simulink library "SimCoreLib"  (R2016b)
settings: Solver=VariableStepAuto  StartTime=0.0  StopTime=10.0  RelTol=1e-3
values from neighbouring files (symbols this model uses):
  Env =     [UAV_modelconfig.mat]
undefined symbols (not defined in the file or in its folder): HDBK, Light, MIL, Sim
undefined symbols (not defined in the file): AC, TrimCondition
libraries: OpenFlightUtilLib x18, SimCoreLib x7, aerolibwind2 x2, aerolib6dofsys x2, aerolibatmos2 x1, aerolibutil x1, aerolib6dof2 x1, aerolibgravity2 x1, aerolibobsolete x1, simulink x1
settings Model: Creator=UAVLAB  LastModifiedBy=rega0051

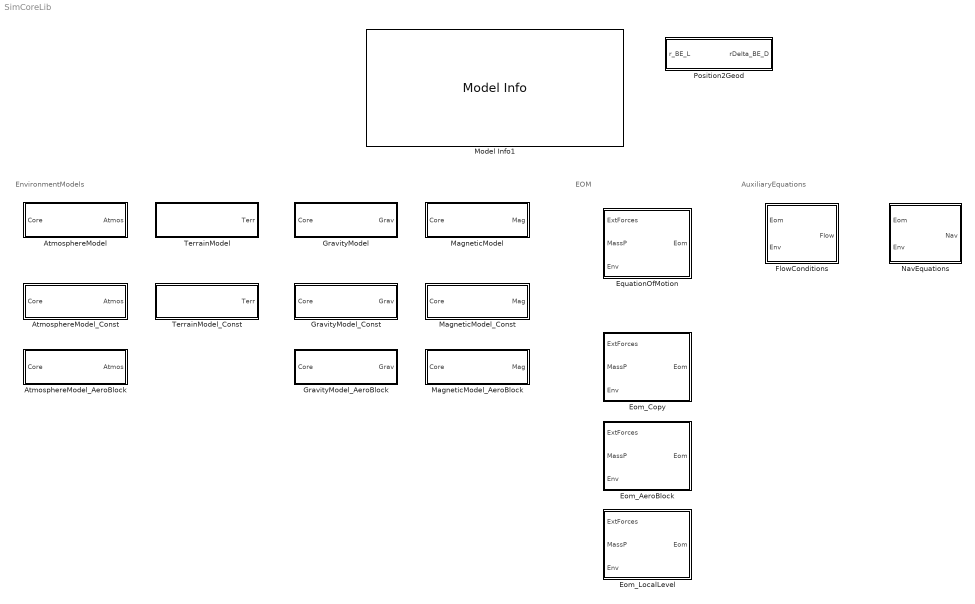
== system SimCoreLib ==
  note: EnvironmentModels
  note: EOM
  note: AuxiliaryEquations
  AtmosphereModel : Subsystem  BlockChoice=AtmosphereModel_AeroBlock
      settings: AttributesFormatString=%<BlockChoice>  TemplateBlock=self  MemberBlocks=AtmosphereModel_AeroBlock,AtmosphereModel_Const
  AtmosphereModel_AeroBlock : Subsystem
  AtmosphereModel_Const : Subsystem
  Eom_AeroBlock : Subsystem  mask(6DoF EoM (Body Axis)){units=Metric (MKS), mtype=Fixed, rep=Euler Angles, xme_0=TrimCondition.InertialIni, Vm_0=TrimCondition.VelocitiesIni, eul_0=TrimCondition.AttitudeIni, pm_0=TrimCondition.RatesIni, mass_0=AC.MassP.mass_kg, mass_e=0.5, mass_f=2.0, inertia=AC.MassP.I_B_kgm2, inertia_e=eye(3), inertia_f=2*eye(3), k_quat=1.0}
      mask prompts: mtype "Mass type:"; rep "Representation:"; xme_0 "Initial position in inertial axes [Xe,Ye,Ze]:"; Vm_0 "Initial velocity in body axes [U,v,w]:"; eul_0 "Initial Euler orientation [roll, pitch, yaw]:"; pm_0 "Initial body rotation rates [p,q,r]:"; mass_0 "Initial mass:"; mass_e "Empty mass:"; mass_f "Full mass:"; inertia_e "Empty inertia matrix:"; inertia_f "Full inertia matrix:"; k_quat "Gain for quaternion normalization:"
      mask help:
      | Integrate the six-degrees-of-freedom equations of motion in body axis.
      |
      | This block has been modified from the original Aerospace Blockset
      | implementation. The inertial position vector (Xe) is no longer computed.
      | The original block did not have a way to add steady state winds to the
      | inertial velocities (Ve) prior to integrating to get Xe. Therefore, this
      | step is performed in the Auxiliary Equations block.
      mask Help: eval('asbhelp(''sixdof_euler_angles'')');
      mask TypeOptions units: Metric (MKS) | English (Velocity in ft/s) | English (Velocity in kts)
      mask TypeOptions mtype: Fixed | Simple Variable | Custom Variable
      mask Callback mtype: aeroicon('aeroblk6dofbody');
      mask TypeOptions rep: Euler Angles | Quaternion
      mask Callback rep: aeroicon('aeroblk6dofbody');
  Eom_Copy : Subsystem
  Eom_LocalLevel : Subsystem
      settings: MinAlgLoopOccurrences=on
  EquationOfMotion : Subsystem  BlockChoice=Eom_AeroBlock
      settings: AttributesFormatString=%<BlockChoice>  TemplateBlock=self  MemberBlocks=Eom_AeroBlock,Eom_Copy,Eom_LocalLevel
  FlowConditions : Subsystem
  GravityModel : Subsystem  BlockChoice=GravityModel_AeroBlock
      settings: AttributesFormatString=%<BlockChoice>  TemplateBlock=self  MemberBlocks=GravityModel_AeroBlock,GravityModel_Const
  GravityModel_AeroBlock : Subsystem
  GravityModel_Const : Subsystem
  MagneticModel : Subsystem  BlockChoice=MagneticModel_AeroBlock
      settings: AttributesFormatString=%<BlockChoice>  TemplateBlock=self  MemberBlocks=MagneticModel_AeroBlock,MagneticModel_Const
  MagneticModel_AeroBlock : Subsystem
  MagneticModel_Const : Subsystem
  Model Info1 : simulink/Model-Wide Utilities/Model Info  Frame=on  DisplayStringWithTags=|  HorizontalTextAlignment=Left  LeftAlignmentValue=0.02  SourceBlockDiagram=SimCoreLib  TagMaxNumber=20
      | MODEL INFORMATION
      | Simulation Core Library (%<ModelName>)
      | 
      | University of Minnesota
      | Aerospace Engineering and Mechanics
      | Copyright 2017 Regents of the University of Minnesota. All rights reserved.
      | 
      | == Update Info ==
      | Last modified by %<LastModifiedBy> on %<LastModificationDate>
  NavEquations : Subsystem
  Position2Geod : Subsystem
  TerrainModel : Subsystem  BlockChoice=TerrainModel_Const
      settings: AttributesFormatString=%<BlockChoice>  TemplateBlock=self  MemberBlocks=TerrainModel_Const
  TerrainModel_Const : Subsystem

== system SimCoreLib/AtmosphereModel ==
  Core : Inport
  AtmosphereModel_AeroBlock : SimCoreLib/AtmosphereModel_AeroBlock
  Atmos : Outport
  wires:
  Core/1 -> AtmosphereModel_AeroBlock/1
  AtmosphereModel_AeroBlock/1 -> Atmos/1

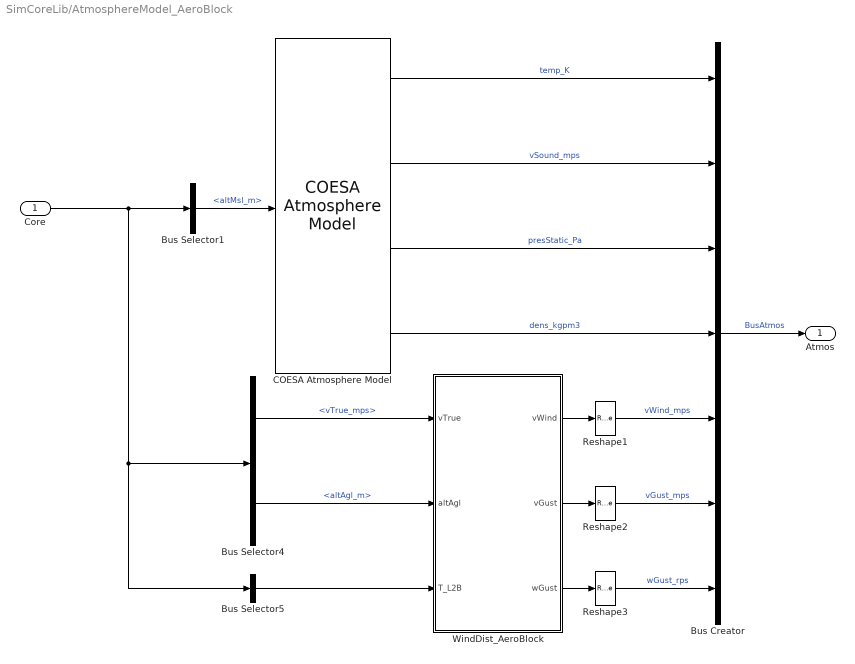
== system SimCoreLib/AtmosphereModel_AeroBlock ==
  Core : Inport
  Bus Creator : BusCreator  Inputs=7  OutDataTypeStr=Bus: BusAtmos
      settings: AttributesFormatString=%<OutDataTypeStr>
  Bus Selector1 : BusSelector  OutputSignals=BusAux.BusNav.altMsl_m
  Bus Selector4 : BusSelector  OutputSignals=BusAux.BusFlow.vTrue_mps,BusAux.BusNav.altAgl_m
  Bus Selector5 : BusSelector  OutputSignals=BusEom.T_L2B  OutputAsBus=on
  COESA Atmosphere Model : aerolibatmos2/COESA Atmosphere Model  units=Metric (MKS)  spec=1976 COESA-extended U.S. Standard Atmosphere  model=Profile  profile_var=High temperature  profile_percent=1%  profile_alt=5 km (16404 ft)  envelope_var=High temperature  envelope_percent=1%  action=Warning
  Reshape1 : Reshape  OutputDimensionality=Column vector (2-D)  OutputDimensions=[3,1]
  Reshape2 : Reshape  OutputDimensionality=Column vector (2-D)  OutputDimensions=[3,1]
  Reshape3 : Reshape  OutputDimensionality=Column vector (2-D)  OutputDimensions=[3,1]
  WindDist_AeroBlock : Subsystem
  Atmos : Outport
  wires:
  Reshape3/1 -> Bus Creator/7  "wGust_rps"
  Reshape2/1 -> Bus Creator/6  "vGust_mps"
  Reshape1/1 -> Bus Creator/5  "vWind_mps"
  WindDist_AeroBlock/1(vWind) -> Reshape1/1
  WindDist_AeroBlock/3(wGust) -> Reshape3/1
  WindDist_AeroBlock/2(vGust) -> Reshape2/1
  Bus Selector1/1 -> COESA Atmosphere Model/1  "<altMsl_m>"
  Bus Selector5/1 -> WindDist_AeroBlock/3(T_L2B)
  Bus Selector4/1 -> WindDist_AeroBlock/1(vTrue)  "<vTrue_mps>"
  COESA Atmosphere Model/4 -> Bus Creator/4  "dens_kgpm3"
  COESA Atmosphere Model/3 -> Bus Creator/3  "presStatic_Pa"
  COESA Atmosphere Model/2 -> Bus Creator/2  "vSound_mps"
  COESA Atmosphere Model/1 -> Bus Creator/1  "temp_K"
  Core/1 -> Bus Selector1/1, Bus Selector4/1, Bus Selector5/1
  Bus Creator/1 -> Atmos/1  "BusAtmos"
  Bus Selector4/2 -> WindDist_AeroBlock/2(altAgl)  "<altAgl_m>"

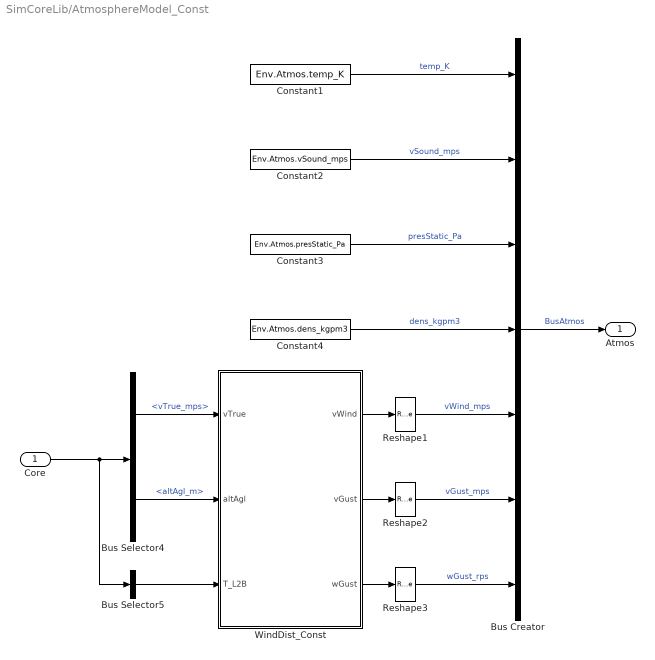
== system SimCoreLib/AtmosphereModel_Const ==
  Core : Inport
  Bus Creator : BusCreator  Inputs=7  OutDataTypeStr=Bus: BusAtmos
      settings: AttributesFormatString=%<OutDataTypeStr>
  Bus Selector4 : BusSelector  OutputSignals=BusAux.BusFlow.vTrue_mps,BusAux.BusNav.altAgl_m
  Bus Selector5 : BusSelector  OutputSignals=BusEom.T_L2B  OutputAsBus=on
  Constant1 : Constant  Value=Env.Atmos.temp_K
      settings: AttributesFormatString=%<Value>
  Constant2 : Constant  Value=Env.Atmos.vSound_mps
      settings: AttributesFormatString=%<Value>
  Constant3 : Constant  Value=Env.Atmos.presStatic_Pa
      settings: AttributesFormatString=%<Value>
  Constant4 : Constant  Value=Env.Atmos.dens_kgpm3
      settings: AttributesFormatString=%<Value>
  Reshape1 : Reshape  OutputDimensionality=Column vector (2-D)  OutputDimensions=[3,1]
  Reshape2 : Reshape  OutputDimensionality=Column vector (2-D)  OutputDimensions=[3,1]
  Reshape3 : Reshape  OutputDimensionality=Column vector (2-D)  OutputDimensions=[3,1]
  WindDist_Const : Subsystem
      settings: MinAlgLoopOccurrences=on
  Atmos : Outport
  wires:
  Reshape3/1 -> Bus Creator/7  "wGust_rps"
  Reshape2/1 -> Bus Creator/6  "vGust_mps"
  Reshape1/1 -> Bus Creator/5  "vWind_mps"
  Bus Creator/1 -> Atmos/1  "BusAtmos"
  Core/1 -> Bus Selector5/1, Bus Selector4/1
  Constant1/1 -> Bus Creator/1  "temp_K"
  WindDist_Const/1(vWind) -> Reshape1/1
  WindDist_Const/3(wGust) -> Reshape3/1
  Constant2/1 -> Bus Creator/2  "vSound_mps"
  Constant3/1 -> Bus Creator/3  "presStatic_Pa"
  WindDist_Const/2(vGust) -> Reshape2/1
  Constant4/1 -> Bus Creator/4  "dens_kgpm3"
  Bus Selector4/1 -> WindDist_Const/1(vTrue)  "<vTrue_mps>"
  Bus Selector4/2 -> WindDist_Const/2(altAgl)  "<altAgl_m>"
  Bus Selector5/1 -> WindDist_Const/3(T_L2B)

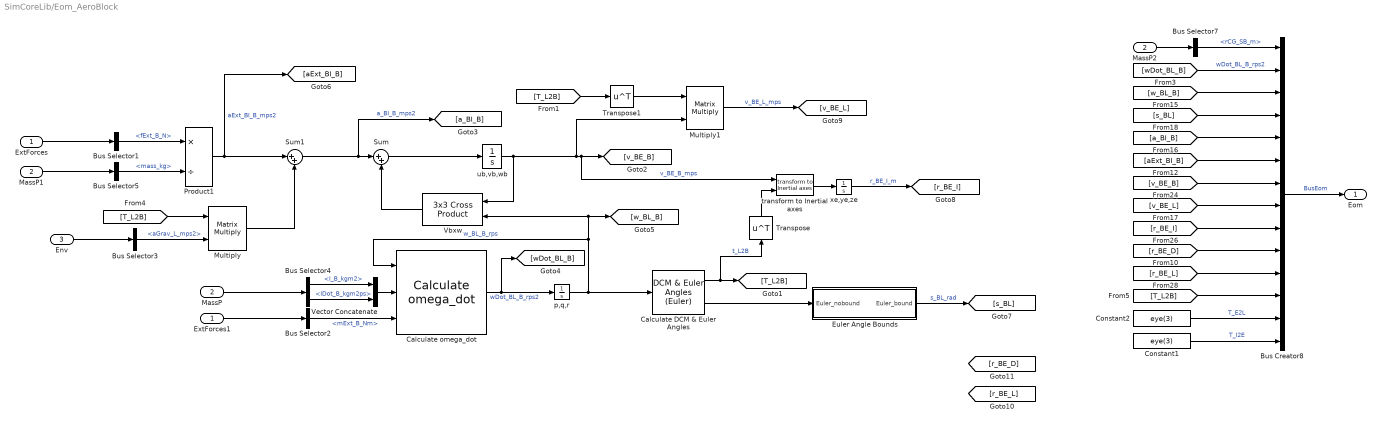
== system SimCoreLib/Eom_AeroBlock ==
  ExtForces : Inport
  MassP : Inport  Port=2
  Env : Inport  Port=3
  Bus Selector1 : BusSelector  OutputSignals=fExt_B_N
  Bus Selector2 : BusSelector  OutputSignals=mExt_B_Nm
  Bus Selector3 : BusSelector  OutputSignals=BusGrav.aGrav_L_mps2
  Bus Selector4 : BusSelector  OutputSignals=I_B_kgm2,IDot_B_kgm2ps
  Bus Selector5 : BusSelector  OutputSignals=mass_kg
  Bus Selector7 : BusSelector  OutputSignals=rCG_SB_m
  Bus Creator8 : BusCreator  Inputs=14  OutDataTypeStr=Bus: BusEom
      settings: AttributesFormatString=%<OutDataTypeStr>
  Calculate DCM & Euler Angles : aerolib6dofsys/DCM & Euler Angles (Euler)  SystemSampleTime=-1
  Calculate omega_dot : aerolib6dofsys/Calculate omega_dot  SystemSampleTime=-1
  Constant1 : Constant  Value=eye(3)
      settings: AttributesFormatString=%<Value>
  Constant2 : Constant  Value=eye(3)
      settings: AttributesFormatString=%<Value>
  Euler Angle Bounds : Subsystem
  ExtForces1 : InportShadow
  MassP1 : InportShadow  Port=2
  MassP2 : InportShadow  Port=2
  Multiply : Product  Multiplication=Matrix(*)  SaturateOnIntegerOverflow=on  InputSameDT=on  OutDataTypeStr=Inherit: Same as first input
  Multiply1 : Product  Multiplication=Matrix(*)  SaturateOnIntegerOverflow=on  InputSameDT=on  OutDataTypeStr=Inherit: Same as first input
  Product1 : Product  Inputs=*/  SaturateOnIntegerOverflow=on  OutDataTypeStr=Inherit: Same as first input
  Sum : Sum  Inputs=|++  SaturateOnIntegerOverflow=on
  Sum1 : Sum  Inputs=|++  SaturateOnIntegerOverflow=on
  Transpose : Math  Operator=transpose  SaturateOnIntegerOverflow=on
  Transpose1 : Math  Operator=transpose  SaturateOnIntegerOverflow=on
  Vbxw : aerolibutil/3x3 Cross Product
  Vector Concatenate : Concatenate  Mode=Multidimensional array
  "p,q,r " : Integrator  InitialCondition=pm_0
  "transform to Inertial axes " : aerolib6dof2/6DOF (Euler Angles)/transform to Inertial axes   SystemSampleTime=-1
  ub,vb,wb : Integrator  InitialCondition=convvel(Vm_0,'m/s','m/s')
  xe,ye,ze : Integrator  InitialCondition=xme_0
  Eom : Outport  OutDataTypeStr=Bus: BusEom
  wires:
  Multiply1/1 -> [v_BE_L]  "v_BE_L_mps"
  [T_L2B] -> Transpose1/1
  Transpose1/1 -> Multiply1/1
  xe,ye,ze/1 -> [r_BE_I]  "r_BE_I_m"
  "transform to Inertial axes "/1 -> xe,ye,ze/1
  Transpose/1 -> "transform to Inertial axes "/2
  Bus Creator8/1 -> Eom/1  "BusEom"
  [T_L2B] -> Bus Creator8/12
  [s_BL] -> Bus Creator8/4
  [a_BI_B] -> Bus Creator8/5
  [r_BE_D] -> Bus Creator8/10
  [w_BL_B] -> Bus Creator8/3
  [aExt_BI_B] -> Bus Creator8/6
  [v_BE_L] -> Bus Creator8/8
  [r_BE_L] -> Bus Creator8/11
  MassP2/1 -> Bus Selector7/1
  Bus Selector7/1 -> Bus Creator8/1  "<rCG_SB_m>"
  [v_BE_B] -> Bus Creator8/7
  [r_BE_I] -> Bus Creator8/9
  Constant1/1 -> Bus Creator8/14  "T_I2E"
  Constant2/1 -> Bus Creator8/13  "T_E2L"
  [wDot_BL_B] -> Bus Creator8/2  "wDot_BL_B_rps2"
  Product1/1 -> Sum1/1, [aExt_BI_B]  "aExt_BI_B_mps2"
  Bus Selector5/1 -> Product1/2  "<mass_kg>"
  MassP1/1 -> Bus Selector5/1
  Vector Concatenate/1 -> Calculate omega_dot/2
  Bus Selector4/1 -> Vector Concatenate/1  "<I_B_kgm2>"
  Bus Selector4/2 -> Vector Concatenate/2  "<IDot_B_kgm2ps>"
  MassP/1 -> Bus Selector4/1
  Bus Selector2/1 -> Calculate omega_dot/3  "<mExt_B_Nm>"
  ExtForces1/1 -> Bus Selector2/1
  Env/1 -> Bus Selector3/1
  Bus Selector3/1 -> Multiply/2  "<aGrav_L_mps2>"
  [T_L2B] -> Multiply/1
  Multiply/1 -> Sum1/2
  Bus Selector1/1 -> Product1/1  "<fExt_B_N>"
  ExtForces/1 -> Bus Selector1/1
  Euler Angle Bounds/1(Euler_bound) -> [s_BL]  "s_BL_rad"
  Calculate DCM & Euler Angles/2 -> Euler Angle Bounds/1(Euler_nobound)
  ub,vb,wb/1 -> Vbxw/1, [v_BE_B], "transform to Inertial axes "/1, Multiply1/2  "v_BE_B_mps"
  Vbxw/1 -> Sum/2
  Sum/1 -> ub,vb,wb/1
  "p,q,r "/1 -> Calculate DCM & Euler Angles/1, Vbxw/2, [w_BL_B], Calculate omega_dot/1  "w_BL_B_rps"
  Sum1/1 -> Sum/1, [a_BI_B]  "a_BI_B_mps2"
  Calculate DCM & Euler Angles/1 -> [T_L2B], Transpose/1  "t_L2B"
  Calculate omega_dot/1 -> "p,q,r "/1, [wDot_BL_B]  "wDot_BL_B_rps2"

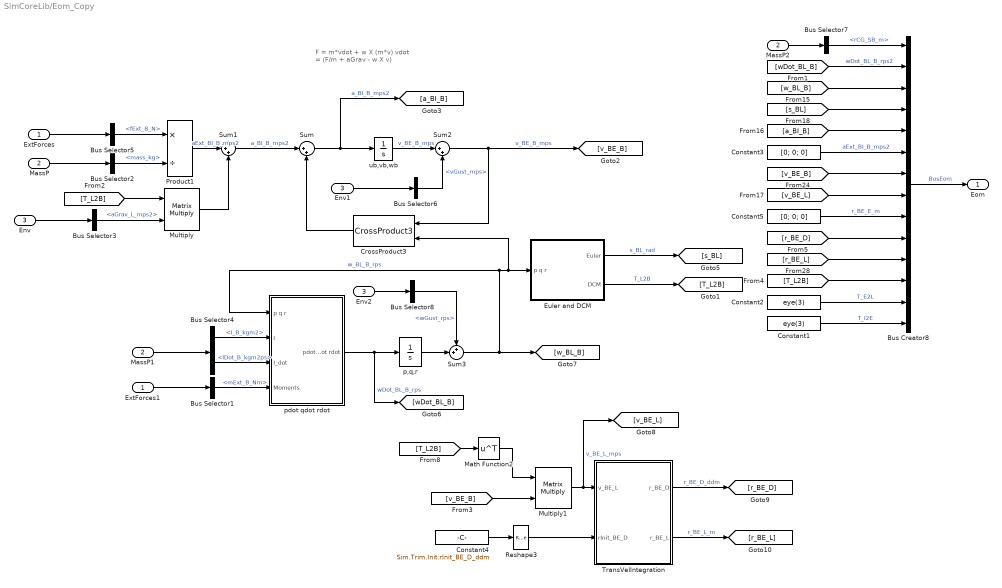
== system SimCoreLib/Eom_Copy ==
  note: F = m*vdot + w X (m*v)
      | vdot = (F/m + aGrav - w X v)
  ExtForces : Inport
  MassP : Inport  Port=2
  Env : Inport  Port=3
  Bus Selector1 : BusSelector  OutputSignals=mExt_B_Nm
  Bus Selector2 : BusSelector  OutputSignals=mass_kg
  Bus Selector3 : BusSelector  OutputSignals=BusGrav.aGrav_L_mps2
  Bus Selector4 : BusSelector  OutputSignals=I_B_kgm2,IDot_B_kgm2ps
  Bus Selector5 : BusSelector  OutputSignals=fExt_B_N
  Bus Selector6 : BusSelector  OutputSignals=BusAtmos.vGust_mps
  Bus Selector7 : BusSelector  OutputSignals=rCG_SB_m
  Bus Selector8 : BusSelector  OutputSignals=BusAtmos.wGust_rps
  Bus Creator8 : BusCreator  Inputs=14  OutDataTypeStr=Bus: BusEom
      settings: AttributesFormatString=%<OutDataTypeStr>
  Constant1 : Constant  Value=eye(3)
      settings: AttributesFormatString=%<Value>
  Constant2 : Constant  Value=eye(3)
      settings: AttributesFormatString=%<Value>
  Constant3 : Constant  Value=[0; 0; 0]
      settings: AttributesFormatString=%<Value>
  Constant4 : Constant  Value=Sim.Trim.Init.rInit_BE_D_ddm
      settings: AttributesFormatString=%<Value>
  Constant5 : Constant  Value=[0; 0; 0]
      settings: AttributesFormatString=%<Value>
  CrossProduct3 : OpenFlightUtilLib/Math/CrossProduct3
  Env1 : InportShadow  Port=3
  Env2 : InportShadow  Port=3
  Euler and DCM : Subsystem
  ExtForces1 : InportShadow
  MassP1 : InportShadow  Port=2
  MassP2 : InportShadow  Port=2
  Math Function2 : Math  Operator=transpose  SaturateOnIntegerOverflow=on
  Multiply : Product  Multiplication=Matrix(*)  SaturateOnIntegerOverflow=on  InputSameDT=on  OutDataTypeStr=Inherit: Same as first input
  Multiply1 : Product  Multiplication=Matrix(*)  SaturateOnIntegerOverflow=on  InputSameDT=on  OutDataTypeStr=Inherit: Same as first input
  Product1 : Product  Inputs=*/  SaturateOnIntegerOverflow=on  OutDataTypeStr=Inherit: Same as first input
  Reshape3 : Reshape  OutputDimensionality=Column vector (2-D)  OutputDimensions=[3,1]
  Sum : Sum  Inputs=|++  SaturateOnIntegerOverflow=on
  Sum1 : Sum  Inputs=|++  SaturateOnIntegerOverflow=on
  Sum2 : Sum  Inputs=|++
  Sum3 : Sum  Inputs=++|
  TransVelIntegration : Subsystem
  "p,q,r " : Integrator  InitialCondition=Sim.Trim.Init.wInit_BL_B_rps  ContinuousStateAttributes='wState_BI_B_rps'
  pdot qdot rdot : Subsystem
  ub,vb,wb : Integrator  ContinuousStateAttributes='vState_BI_B_mps'
  Eom : Outport  OutDataTypeStr=Bus: BusEom
  wires:
  "p,q,r "/1 -> Sum3/2
  Env2/1 -> Bus Selector8/1
  Bus Selector8/1 -> Sum3/1  "<wGust_rps>"
  ub,vb,wb/1 -> Sum2/1  "v_BE_B_mps"
  Bus Selector6/1 -> Sum2/2  "<vGust_mps>"
  Env1/1 -> Bus Selector6/1
  Constant3/1 -> Bus Creator8/6  "aExt_BI_B_mps2"
  Constant5/1 -> Bus Creator8/9  "r_BE_E_m"
  [wDot_BL_B] -> Bus Creator8/2  "wDot_BL_B_rps2"
  Constant2/1 -> Bus Creator8/13  "T_E2L"
  Constant1/1 -> Bus Creator8/14  "T_I2E"
  TransVelIntegration/2(r_BE_L) -> [r_BE_L]  "r_BE_L_m"
  TransVelIntegration/1(r_BE_D) -> [r_BE_D]  "r_BE_D_ddm"
  [v_BE_B] -> Multiply1/2
  Multiply1/1 -> TransVelIntegration/1(v_BE_L), [v_BE_L]  "v_BE_L_mps"
  Math Function2/1 -> Multiply1/1
  [T_L2B] -> Math Function2/1
  Reshape3/1 -> TransVelIntegration/2(rInit_BE_D)
  Constant4/1 -> Reshape3/1
  Euler and DCM/1(Euler) -> [s_BL]  "s_BL_rad"
  [v_BE_B] -> Bus Creator8/7
  Bus Selector7/1 -> Bus Creator8/1  "<rCG_SB_m>"
  MassP2/1 -> Bus Selector7/1
  [r_BE_L] -> Bus Creator8/11
  [v_BE_L] -> Bus Creator8/8
  [w_BL_B] -> Bus Creator8/3
  [r_BE_D] -> Bus Creator8/10
  [a_BI_B] -> Bus Creator8/5
  [s_BL] -> Bus Creator8/4
  [T_L2B] -> Bus Creator8/12
  Bus Creator8/1 -> Eom/1  "BusEom"
  ExtForces1/1 -> Bus Selector1/1
  MassP1/1 -> Bus Selector4/1
  Multiply/1 -> Sum1/2
  [T_L2B] -> Multiply/1
  Bus Selector3/1 -> Multiply/2  "<aGrav_L_mps2>"
  Env/1 -> Bus Selector3/1
  Bus Selector2/1 -> Product1/2  "<mass_kg>"
  MassP/1 -> Bus Selector2/1
  Bus Selector1/1 -> pdot qdot rdot/4(Moments)  "<mExt_B_Nm>"
  Bus Selector5/1 -> Product1/1  "<fExt_B_N>"
  ExtForces/1 -> Bus Selector5/1
  Product1/1 -> Sum1/1  "aExt_BI_B_mps2"
  pdot qdot rdot/1(pdot qdot rdot) -> "p,q,r "/1, [wDot_BL_B]  "wDot_BL_B_rps"
  Sum3/1 -> pdot qdot rdot/1(p q r), CrossProduct3/2, Euler and DCM/1("p q r "), [w_BL_B]  "w_BL_B_rps"
  CrossProduct3/1 -> Sum/2
  Sum/1 -> ub,vb,wb/1, [a_BI_B]  "a_BI_B_mps2"
  Sum1/1 -> Sum/1  "a_BI_B_mps2"
  Euler and DCM/2(DCM) -> [T_L2B]  "T_L2B"
  Sum2/1 -> [v_BE_B], CrossProduct3/1  "v_BE_B_mps"
  Bus Selector4/2 -> pdot qdot rdot/3(I_dot)  "<IDot_B_kgm2ps>"
  Bus Selector4/1 -> pdot qdot rdot/2(I)  "<I_B_kgm2>"

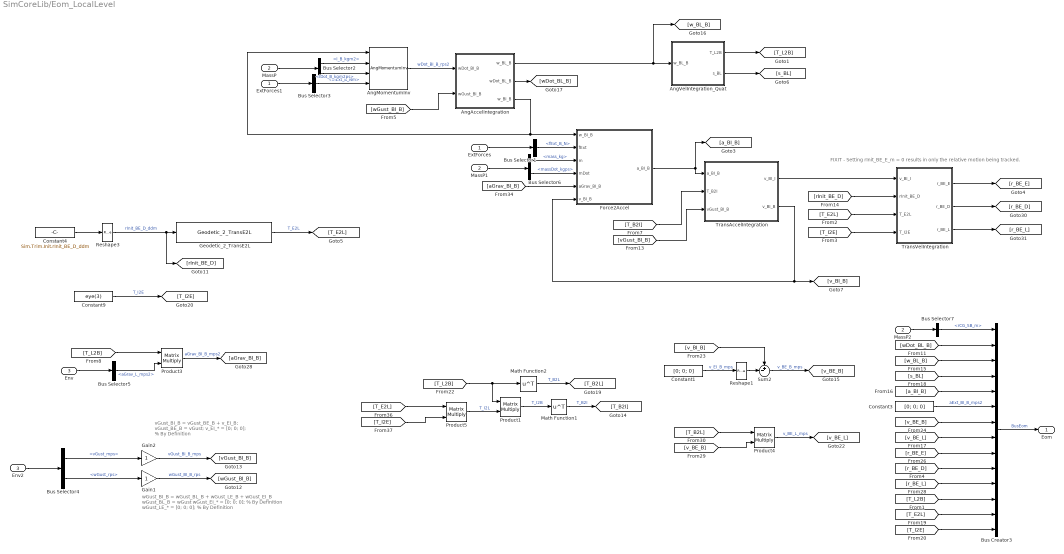
== system SimCoreLib/Eom_LocalLevel ==
  note: wGust_BI_B = wGust_BL_B + wGust_LE_B + wGust_EI_B
      | wGust_BL_B = wGust
      | wGust_EI_* = [0; 0; 0]; % By Definition
      | wGust_LE_* = [0; 0; 0]; % By Definition
  note: vGust_BI_B = vGust_BE_B + v_EI_B;
      | vGust_BE_B = vGust;
      | v_EI_* = [0; 0; 0]; % By Definition
  note: FIXIT - Setting rInit_BE_E_m = 0 results in only the relative motion being tracked.
  ExtForces : Inport
  MassP : Inport  Port=2
  Env : Inport  Port=3  OutDataTypeStr=Bus: BusEnv
  AngAccelIntegration : Subsystem
  AngMomentumInv : OpenFlightUtilLib/Kinematics and Dynamics/AngMomentumInv
  AngVelIntegration_Quat : Subsystem
  Bus Selector1 : BusSelector  OutputSignals=fExt_B_N
  Bus Selector2 : BusSelector  OutputSignals=I_B_kgm2,IDot_B_kgm2ps
  Bus Selector3 : BusSelector  OutputSignals=mExt_B_Nm
  Bus Selector4 : BusSelector  OutputSignals=BusAtmos.vGust_mps,BusAtmos.wGust_rps
  Bus Selector5 : BusSelector  OutputSignals=BusGrav.aGrav_L_mps2
  Bus Selector6 : BusSelector  OutputSignals=mass_kg,massDot_kgps
  Bus Selector7 : BusSelector  OutputSignals=rCG_SB_m
  Bus Creator3 : BusCreator  Inputs=14  OutDataTypeStr=Bus: BusEom
      settings: AttributesFormatString=%<OutDataTypeStr>
  Constant1 : Constant  Value=[0; 0; 0]
      settings: AttributesFormatString=%<Value>
  Constant3 : Constant  Value=[0; 0; 0]
      settings: AttributesFormatString=%<Value>
  Constant4 : Constant  Value=Sim.Trim.Init.rInit_BE_D_ddm
      settings: AttributesFormatString=%<Value>
  Constant9 : Constant  Value=eye(3)
      settings: AttributesFormatString=%<Value>
  Env2 : InportShadow  Port=3  OutDataTypeStr=Bus: BusEnv
  ExtForces1 : InportShadow
  Force2Accel : Subsystem
  Gain1 : Gain
  Gain2 : Gain
  Geodetic_2_TransE2L : OpenFlightUtilLib/Transformations/Geodetic_2_TransE2L
  MassP1 : InportShadow  Port=2
  MassP2 : InportShadow  Port=2
  Math Function1 : Math  Operator=transpose  SaturateOnIntegerOverflow=on
  Math Function2 : Math  Operator=transpose  SaturateOnIntegerOverflow=on
  Product{1,3..5} (4 alike) : Product  Inputs=**  Multiplication=Matrix(*)  RndMeth=Zero
  Reshape1 : Reshape  OutputDimensionality=Column vector (2-D)  OutputDimensions=[3,1]
  Reshape3 : Reshape  OutputDimensionality=Column vector (2-D)  OutputDimensions=[3,1]
  Sum2 : Sum  Inputs=+-|
  TransAccelIntegration : Subsystem
  TransVelIntegration : Subsystem
  Eom : Outport
  wires:
  [T_I2E] -> TransVelIntegration/4(T_I2E)
  Constant4/1 -> Reshape3/1
  Constant3/1 -> Bus Creator3/6  "aExt_BI_B_mps2"
  TransAccelIntegration/2(v_BI_B) -> [v_BI_B], Force2Accel/6(v_BI_B)
  AngAccelIntegration/3(w_BI_B) -> Force2Accel/1(w_BI_B), AngMomentumInv/1
  Reshape1/1 -> Sum2/2
  Math Function2/1 -> [T_B2L]  "T_B2L"
  [v_BI_B] -> Sum2/1
  Constant1/1 -> Reshape1/1  "v_EI_B_mps"
  Sum2/1 -> [v_BE_B]  "v_BE_B_mps"
  [T_E2L] -> TransVelIntegration/3(T_E2L)
  [r_BE_E] -> Bus Creator3/9
  [v_BE_B] -> Bus Creator3/7
  [vGust_BI_B] -> TransAccelIntegration/3(vGust_BI_B)
  Gain1/1 -> [wGust_BI_B]  "wGust_BI_B_rps"
  Gain2/1 -> [vGust_BI_B]  "vGust_BI_B_mps"
  Bus Selector4/2 -> Gain1/1  "<wGust_rps>"
  Env2/1 -> Bus Selector4/1
  [wGust_BI_B] -> AngAccelIntegration/2(wGust_BI_B)
  Bus Selector7/1 -> Bus Creator3/1  "<rCG_SB_m>"
  MassP2/1 -> Bus Selector7/1
  [T_E2L] -> Product5/1
  [T_I2E] -> Product5/2
  [rInit_BE_D] -> TransVelIntegration/2(rInit_BE_D)
  TransVelIntegration/3(r_BE_L) -> [r_BE_L]
  TransVelIntegration/2(r_BE_D) -> [r_BE_D]
  AngAccelIntegration/2(wDot_BL_B) -> [wDot_BL_B]
  [aGrav_BI_B] -> Force2Accel/5(aGrav_BI_B)
  Bus Selector4/1 -> Gain2/1  "<vGust_mps>"
  Product5/1 -> Product1/2  "T_I2L"
  [T_B2L] -> Product4/1
  [v_BE_B] -> Product4/2
  [r_BE_L] -> Bus Creator3/11
  Product4/1 -> [v_BE_L]  "v_BE_L_mps"
  [T_L2B] -> Product1/1, Math Function2/1
  Constant9/1 -> [T_I2E]  "T_I2E"
  Geodetic_2_TransE2L/1 -> [T_E2L]  "T_E2L"
  [T_I2E] -> Bus Creator3/14
  [T_E2L] -> Bus Creator3/13
  AngAccelIntegration/1(w_BL_B) -> [w_BL_B], AngVelIntegration_Quat/1(w_BL_B)
  [v_BE_L] -> Bus Creator3/8
  [wDot_BL_B] -> Bus Creator3/2
  [w_BL_B] -> Bus Creator3/3
  [r_BE_D] -> Bus Creator3/10
  [a_BI_B] -> Bus Creator3/5
  [s_BL] -> Bus Creator3/4
  MassP1/1 -> Bus Selector6/1
  Bus Selector3/1 -> AngMomentumInv/4  "<mExt_B_Nm>"
  Bus Selector2/2 -> AngMomentumInv/3  "<IDot_B_kgm2ps>"
  Bus Selector2/1 -> AngMomentumInv/2  "<I_B_kgm2>"
  AngMomentumInv/1 -> AngAccelIntegration/1(wDot_BI_B)  "wDot_BI_B_rps2"
  Force2Accel/1(a_BI_B) -> [a_BI_B], TransAccelIntegration/1(a_BI_B)
  AngVelIntegration_Quat/2(s_BL) -> [s_BL]
  [T_L2B] -> Product3/1
  Bus Selector5/1 -> Product3/2  "<aGrav_L_mps2>"
  Env/1 -> Bus Selector5/1
  ExtForces1/1 -> Bus Selector3/1
  MassP/1 -> Bus Selector2/1
  [T_L2B] -> Bus Creator3/12
  Bus Creator3/1 -> Eom/1  "BusEom"
  Bus Selector1/1 -> Force2Accel/2(fExt)  "<fExt_B_N>"
  ExtForces/1 -> Bus Selector1/1
  AngVelIntegration_Quat/1(T_L2B) -> [T_L2B]
  Product3/1 -> [aGrav_BI_B]  "aGrav_BI_B_mps2"
  Bus Selector6/1 -> Force2Accel/3(m)  "<mass_kg>"
  Bus Selector6/2 -> Force2Accel/4(mDot)  "<massDot_kgps>"
  TransAccelIntegration/1(v_BI_I) -> TransVelIntegration/1(v_BI_I)
  TransVelIntegration/1(r_BE_E) -> [r_BE_E]
  [T_B2I] -> TransAccelIntegration/2(T_B2I)
  Product1/1 -> Math Function1/1  "T_I2B"
  Math Function1/1 -> [T_B2I]  "T_B2I"
  Reshape3/1 -> Geodetic_2_TransE2L/1, [rInit_BE_D]  "rInit_BE_D_ddm"

== system SimCoreLib/EquationOfMotion ==
  ExtForces : Inport
  MassP : Inport  Port=2
  Env : Inport  Port=3
  Eom_AeroBlock : SimCoreLib/Eom_AeroBlock  units=Metric (MKS)  mtype=Fixed  rep=Euler Angles  xme_0=TrimCondition.InertialIni  Vm_0=TrimCondition.VelocitiesIni  eul_0=TrimCondition.AttitudeIni  pm_0=TrimCondition.RatesIni  mass_0=AC.MassP.mass_kg  mass_e=0.5  mass_f=2.0  inertia=AC.MassP.I_B_kgm2  inertia_e=eye(3)  inertia_f=2*eye(3)  k_quat=1.0
  Eom : Outport
  wires:
  ExtForces/1 -> Eom_AeroBlock/1
  MassP/1 -> Eom_AeroBlock/2
  Env/1 -> Eom_AeroBlock/3
  Eom_AeroBlock/1 -> Eom/1

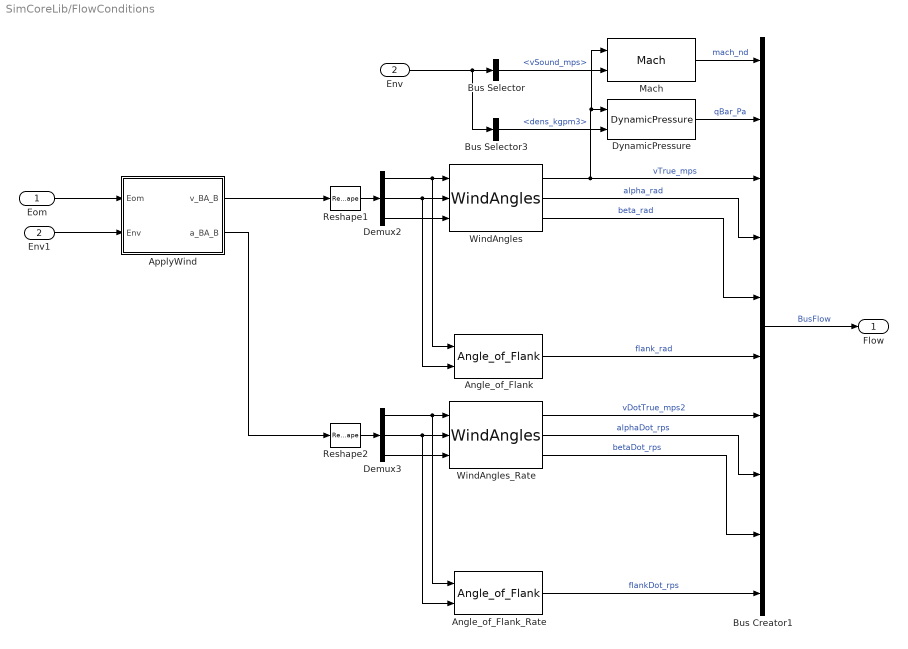
== system SimCoreLib/FlowConditions ==
  Eom : Inport
  Env : Inport  Port=2
  Angle_of_Flank : OpenFlightUtilLib/Air Data/Angle_of_Flank
  Angle_of_Flank_Rate : OpenFlightUtilLib/Air Data/Angle_of_Flank
  ApplyWind : Subsystem
  Bus Creator1 : BusCreator  Inputs=10  OutDataTypeStr=Bus: BusFlow
      settings: InheritFromInputs=off
  Bus Selector : BusSelector  OutputSignals=BusAtmos.vSound_mps
  Bus Selector3 : BusSelector  OutputSignals=BusAtmos.dens_kgpm3
  Demux2 : Demux  Outputs=3
  Demux3 : Demux  Outputs=3
  DynamicPressure : OpenFlightUtilLib/Air Data/DynamicPressure
  Env1 : InportShadow  Port=2
  Mach : OpenFlightUtilLib/Air Data/Mach
  Reshape1 : Reshape  OutputDimensions=[3,1]
  Reshape2 : Reshape  OutputDimensions=[3,1]
  WindAngles : OpenFlightUtilLib/Air Data/WindAngles
  WindAngles_Rate : OpenFlightUtilLib/Air Data/WindAngles
  Flow : Outport
  wires:
  Reshape2/1 -> Demux3/1
  Reshape1/1 -> Demux2/1
  ApplyWind/2(a_BA_B) -> Reshape2/1
  Env1/1 -> ApplyWind/2(Env)
  Eom/1 -> ApplyWind/1(Eom)
  WindAngles_Rate/2 -> Bus Creator1/8  "alphaDot_rps"
  Demux3/2 -> Angle_of_Flank_Rate/2, WindAngles_Rate/2
  WindAngles_Rate/1 -> Bus Creator1/7  "vDotTrue_mps2"
  Demux3/3 -> WindAngles_Rate/3
  Demux3/1 -> Angle_of_Flank_Rate/1, WindAngles_Rate/1
  WindAngles_Rate/3 -> Bus Creator1/9  "betaDot_rps"
  WindAngles/3 -> Bus Creator1/5  "beta_rad"
  Angle_of_Flank/1 -> Bus Creator1/6  "flank_rad"
  Angle_of_Flank_Rate/1 -> Bus Creator1/10  "flankDot_rps"
  Bus Creator1/1 -> Flow/1  "BusFlow"
  WindAngles/2 -> Bus Creator1/4  "alpha_rad"
  Demux2/2 -> Angle_of_Flank/2, WindAngles/2
  Demux2/1 -> Angle_of_Flank/1, WindAngles/1
  WindAngles/1 -> Mach/1, DynamicPressure/1, Bus Creator1/3  "vTrue_mps"
  Demux2/3 -> WindAngles/3
  DynamicPressure/1 -> Bus Creator1/2  "qBar_Pa"
  Bus Selector3/1 -> DynamicPressure/2  "<dens_kgpm3>"
  Env/1 -> Bus Selector3/1, Bus Selector/1
  Bus Selector/1 -> Mach/2  "<vSound_mps>"
  Mach/1 -> Bus Creator1/1  "mach_nd"
  ApplyWind/1(v_BA_B) -> Reshape1/1

== system SimCoreLib/GravityModel ==
  Core : Inport
  GravityModel_AeroBlock : SimCoreLib/GravityModel_AeroBlock
  Grav : Outport
  wires:
  Core/1 -> GravityModel_AeroBlock/1
  GravityModel_AeroBlock/1 -> Grav/1

== system SimCoreLib/GravityModel_AeroBlock ==
  Core : Inport
  Bus Creator : BusCreator  Inputs=1  OutDataTypeStr=Bus: BusGrav
      settings: AttributesFormatString=%<OutDataTypeStr>
  Bus Selector3 : BusSelector  OutputSignals=BusEom.r_BE_D_ddm
  Memory1 : Memory  X0=Sim.Trim.Init.rInit_BE_D_ddm  InheritSampleTime=on  LinearizeMemory=on  LinearizeAsDelay=on
      settings: AttributesFormatString=%<X0>
  Reshape : Reshape  OutputDimensions=3
  Reshape1 : Reshape  OutputDimensionality=Column vector (2-D)  OutputDimensions=[3,1]
  "WGS84 Gravity Model " : aerolibgravity2/WGS84 Gravity Model   model=WGS84 Taylor Series  units=Metric (MKS)  no_atmos=on  precessing=on  jd_loc=off  month=October  day=10  year=2004  no_centrifugal=on  action=Warning
  Grav : Outport
  wires:
  Memory1/1 -> Reshape/1
  Reshape/1 -> "WGS84 Gravity Model "/1
  Reshape1/1 -> Bus Creator/1  "aGrav_L_mps2"
  "WGS84 Gravity Model "/1 -> Reshape1/1
  Bus Selector3/1 -> Memory1/1  "<r_BE_D_ddm>"
  Core/1 -> Bus Selector3/1
  Bus Creator/1 -> Grav/1  "BusGrav"

== system SimCoreLib/GravityModel_Const ==
  Core : Inport
  Bus Creator : BusCreator  Inputs=1  OutDataTypeStr=Bus: BusGrav
      settings: AttributesFormatString=%<OutDataTypeStr>
  Constant : Constant  Value=Env.Grav.aGrav_L_mps2
      settings: AttributesFormatString=%<Value>
  Reshape1 : Reshape  OutputDimensionality=Column vector (2-D)  OutputDimensions=[3,1]
  declination : Terminator
  Grav : Outport
  wires:
  Constant/1 -> Reshape1/1
  Bus Creator/1 -> Grav/1  "BusGrav"
  Core/1 -> declination/1
  Reshape1/1 -> Bus Creator/1  "aGrav_L_mps2"

== system SimCoreLib/MagneticModel ==
  Core : Inport
  MagneticModel_AeroBlock : SimCoreLib/MagneticModel_AeroBlock
  Mag : Outport
  wires:
  Core/1 -> MagneticModel_AeroBlock/1
  MagneticModel_AeroBlock/1 -> Mag/1

== system SimCoreLib/MagneticModel_AeroBlock ==
  Core : Inport
  Bus Creator1 : BusCreator  Inputs=1  OutDataTypeStr=Bus: BusMag
      settings: AttributesFormatString=%<OutDataTypeStr>  InheritFromInputs=off
  Bus Selector3 : BusSelector  OutputSignals=BusEom.r_BE_D_ddm
  Constant1 : Constant  Value=Env.Date.year
      settings: AttributesFormatString=%<Value>
  Demux : Demux  Outputs=3
  Memory1 : Memory  X0=Sim.Trim.Init.rInit_BE_D_ddm  InheritSampleTime=on  LinearizeMemory=on  LinearizeAsDelay=on
      settings: AttributesFormatString=%<X0>
  Reshape1 : Reshape  OutputDimensionality=Column vector (2-D)  OutputDimensions=[3,1]
  World Magnetic Model 2005 : aerolibobsolete/World Magnetic Model 2005  units=Metric (MKS)  time_in=on  month=January  day=1  year=2005  action=None  h_out=off  dec_out=off  inc_out=off  ti_out=off
  Mag : Outport
  wires:
  Memory1/1 -> Demux/1
  Bus Selector3/1 -> Memory1/1  "<r_BE_D_ddm>"
  Reshape1/1 -> Bus Creator1/1  "h_L_nT"
  Core/1 -> Bus Selector3/1
  Demux/1 -> World Magnetic Model 2005/2
  Demux/2 -> World Magnetic Model 2005/3
  Demux/3 -> World Magnetic Model 2005/1
  Constant1/1 -> World Magnetic Model 2005/4
  World Magnetic Model 2005/1 -> Reshape1/1
  Bus Creator1/1 -> Mag/1  "BusMag"

== system SimCoreLib/MagneticModel_Const ==
  Core : Inport
  Bus Creator1 : BusCreator  Inputs=1  OutDataTypeStr=Bus: BusMag
      settings: AttributesFormatString=%<OutDataTypeStr>  InheritFromInputs=off
  Constant : Constant  Value=Env.Mag.h_L_nT
      settings: AttributesFormatString=%<Value>
  Reshape1 : Reshape  OutputDimensionality=Column vector (2-D)  OutputDimensions=[3,1]
  declination : Terminator
  Mag : Outport
  wires:
  Reshape1/1 -> Bus Creator1/1  "h_L_nT"
  Core/1 -> declination/1
  Constant/1 -> Reshape1/1
  Bus Creator1/1 -> Mag/1  "BusMag"

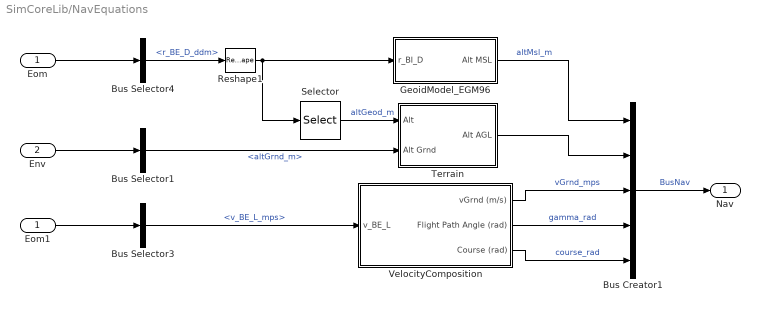
== system SimCoreLib/NavEquations ==
  Eom : Inport
  Env : Inport  Port=2
  Bus Creator1 : BusCreator  Inputs=5  OutDataTypeStr=Bus: BusNav
      settings: AttributesFormatString=%<OutDataTypeStr>  InheritFromInputs=off
  Bus Selector1 : BusSelector  OutputSignals=BusTerr.altGrnd_m
  Bus Selector3 : BusSelector  OutputSignals=v_BE_L_mps
  Bus Selector4 : BusSelector  OutputSignals=r_BE_D_ddm
  Eom1 : InportShadow
  GeoidModel_EGM96 : Subsystem
  Reshape1 : Reshape  OutputDimensions=[3,1]
  Selector : Selector  InputPortWidth=3  IndexOptions=Index vector (dialog)  Indices=3  OutputSizes=1
  Terrain : Subsystem
  VelocityComposition : Subsystem
  Nav : Outport
  wires:
  Reshape1/1 -> Selector/1, GeoidModel_EGM96/1(r_BI_D)
  Bus Selector4/1 -> Reshape1/1  "<r_BE_D_ddm>"
  Bus Selector3/1 -> VelocityComposition/1(v_BE_L)  "<v_BE_L_mps>"
  Eom1/1 -> Bus Selector3/1
  Bus Creator1/1 -> Nav/1  "BusNav"
  GeoidModel_EGM96/1(Alt MSL) -> Bus Creator1/1  "altMsl_m"
  Selector/1 -> Terrain/1(Alt)  "altGeod_m"
  VelocityComposition/1(vGrnd (m/s)) -> Bus Creator1/3  "vGrnd_mps"
  VelocityComposition/2(Flight Path Angle (rad)) -> Bus Creator1/4  "gamma_rad"
  VelocityComposition/3(Course (rad)) -> Bus Creator1/5  "course_rad"
  Eom/1 -> Bus Selector4/1
  Terrain/1(Alt AGL) -> Bus Creator1/2
  Bus Selector1/1 -> Terrain/2(Alt Grnd)  "<altGrnd_m>"
  Env/1 -> Bus Selector1/1

== system SimCoreLib/Position2Geod ==
  r_BE_L : Inport
  Constant1 : Constant  Value=Env.Earth.radiusEquator_m
      settings: AttributesFormatString=%<Value>
  Constant2 : Constant  Value=Env.Earth.radiusPolar_m
      settings: AttributesFormatString=%<Value>
  Demux1 : Demux  Outputs=3
  Gain : Gain  Gain=180/pi
      settings: AttributesFormatString=%<Gain>
  Gain1 : Gain  Gain=-1
      settings: AttributesFormatString=%<Gain>
  Gain2 : Gain  Gain=180/pi
      settings: AttributesFormatString=%<Gain>
  Mux : Mux  Inputs=3
  Product : Product  Inputs=*/
  Product1 : Product  Inputs=*/
  rDelta_BE_D : Outport
  wires:
  Gain1/1 -> Mux/3
  Mux/1 -> rDelta_BE_D/1  "rDelta_BE_D_ddm"
  Demux1/3 -> Gain1/1
  Demux1/1 -> Product/1
  Constant2/1 -> Product/2
  r_BE_L/1 -> Demux1/1
  Gain2/1 -> Mux/1
  Product/1 -> Gain2/1
  Constant1/1 -> Product1/2
  Demux1/2 -> Product1/1
  Product1/1 -> Gain/1
  Gain/1 -> Mux/2

== system SimCoreLib/TerrainModel ==
  TerrainModel_Const : SimCoreLib/TerrainModel_Const
  Terr : Outport
  wires:
  TerrainModel_Const/1 -> Terr/1

== system SimCoreLib/TerrainModel_Const ==
  Bus Creator1 : BusCreator  Inputs=1  OutDataTypeStr=Bus: BusTerr
      settings: AttributesFormatString=%<OutDataTypeStr>
  Constant : Constant  Value=Env.Terr.altGrd_m
      settings: AttributesFormatString=%<Value>
  Terr : Outport
  wires:
  Bus Creator1/1 -> Terr/1  "BusTerr"
  Constant/1 -> Bus Creator1/1  "altGrnd_m"

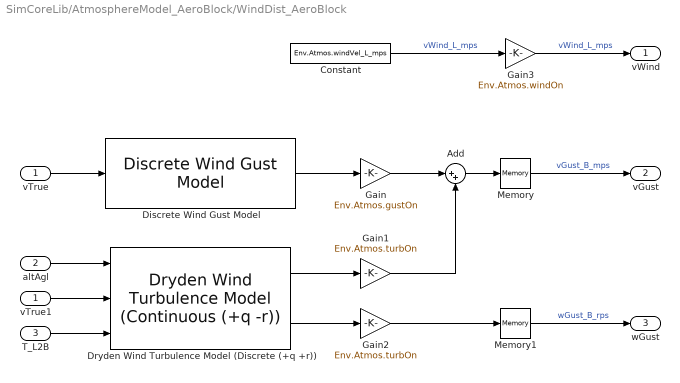
== system SimCoreLib/AtmosphereModel_AeroBlock/WindDist_AeroBlock ==
  vTrue : Inport
  altAgl : Inport  Port=2
  T_L2B : Inport  Port=3
  Add : Sum  Inputs=|++
  Constant : Constant  Value=Env.Atmos.windVel_L_mps
      settings: AttributesFormatString=%<Value>
  Discrete Wind Gust Model : aerolibwind2/Discrete Wind Gust Model  units=Metric (MKS)  Gx=on  Gy=on  Gz=on  t_0=Env.Atmos.gustTimeStart_s  d_m=Env.Atmos.gustLen_m  v_m=Env.Atmos.gustVelMag_B_mps
  Dryden Wind Turbulence Model (Discrete (+q +r)) : aerolibwind2/Dryden Wind Turbulence Model  (Continuous (+q -r))  units=Metric (MKS)  spec=MIL-HDBK-1797B  model=Discrete Dryden (+q +r)  W20=Env.Atmos.windVelMag_mps  Wdeg=Env.Atmos.windVelDir_deg  TurbProb=10^-2 - Light  L_high=762  Wingspan=Env.Atmos.turbSpan_m  ts=Env.Atmos.turbTimeSample_s  Seed=Env.Atmos.turbSeed  T_on=on
  Gain : Gain  Gain=Env.Atmos.gustOn
      settings: AttributesFormatString=%<Gain>
  Gain1 : Gain  Gain=Env.Atmos.turbOn
      settings: AttributesFormatString=%<Gain>
  Gain2 : Gain  Gain=Env.Atmos.turbOn
      settings: AttributesFormatString=%<Gain>
  Gain3 : Gain  Gain=Env.Atmos.windOn
      settings: AttributesFormatString=%<Gain>
  Memory : Memory
  Memory1 : Memory
  vTrue1 : InportShadow
  vWind : Outport
  vGust : Outport  Port=2
  wGust : Outport  Port=3
  wires:
  vTrue/1 -> Discrete Wind Gust Model/1
  Constant/1 -> Gain3/1  "vWind_L_mps"
  Add/1 -> Memory/1
  Discrete Wind Gust Model/1 -> Gain/1
  Dryden Wind Turbulence Model (Discrete (+q +r))/1 -> Gain1/1
  Gain2/1 -> Memory1/1
  Gain3/1 -> vWind/1  "vWind_L_mps"
  Gain/1 -> Add/1
  Gain1/1 -> Add/2
  Dryden Wind Turbulence Model (Discrete (+q +r))/2 -> Gain2/1
  T_L2B/1 -> Dryden Wind Turbulence Model (Discrete (+q +r))/3
  altAgl/1 -> Dryden Wind Turbulence Model (Discrete (+q +r))/1
  vTrue1/1 -> Dryden Wind Turbulence Model (Discrete (+q +r))/2
  Memory/1 -> vGust/1  "vGust_B_mps"
  Memory1/1 -> wGust/1  "wGust_B_rps"

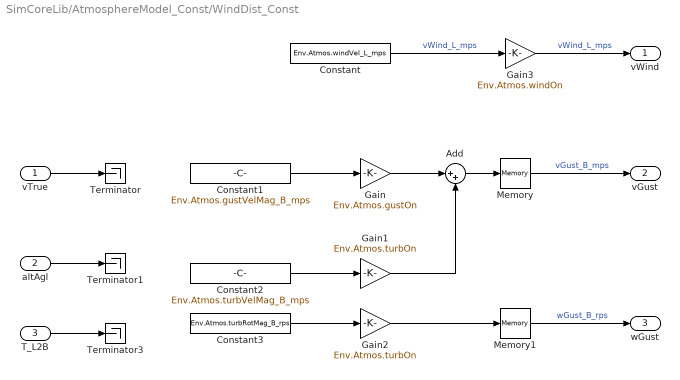
== system SimCoreLib/AtmosphereModel_Const/WindDist_Const ==
  vTrue : Inport
  altAgl : Inport  Port=2
  T_L2B : Inport  Port=3
  Add : Sum  Inputs=|++
  Constant : Constant  Value=Env.Atmos.windVel_L_mps
      settings: AttributesFormatString=%<Value>
  Constant1 : Constant  Value=Env.Atmos.gustVelMag_B_mps
      settings: AttributesFormatString=%<Value>
  Constant2 : Constant  Value=Env.Atmos.turbVelMag_B_mps
      settings: AttributesFormatString=%<Value>
  Constant3 : Constant  Value=Env.Atmos.turbRotMag_B_rps
      settings: AttributesFormatString=%<Value>
  Gain : Gain  Gain=Env.Atmos.gustOn
      settings: AttributesFormatString=%<Gain>
  Gain1 : Gain  Gain=Env.Atmos.turbOn
      settings: AttributesFormatString=%<Gain>
  Gain2 : Gain  Gain=Env.Atmos.turbOn
      settings: AttributesFormatString=%<Gain>
  Gain3 : Gain  Gain=Env.Atmos.windOn
      settings: AttributesFormatString=%<Gain>
  Memory : Memory
  Memory1 : Memory
  Terminator : Terminator
  Terminator1 : Terminator
  Terminator3 : Terminator
  vWind : Outport
  vGust : Outport  Port=2
  wGust : Outport  Port=3
  wires:
  vTrue/1 -> Terminator/1
  Constant/1 -> Gain3/1  "vWind_L_mps"
  Add/1 -> Memory/1
  Constant1/1 -> Gain/1
  Constant2/1 -> Gain1/1
  Gain2/1 -> Memory1/1
  Gain3/1 -> vWind/1  "vWind_L_mps"
  Gain/1 -> Add/1
  Gain1/1 -> Add/2
  Constant3/1 -> Gain2/1
  T_L2B/1 -> Terminator3/1
  altAgl/1 -> Terminator1/1
  Memory/1 -> vGust/1  "vGust_B_mps"
  Memory1/1 -> wGust/1  "wGust_B_rps"

== system SimCoreLib/Eom_AeroBlock/Euler Angle Bounds ==
  Euler_nobound : Inport
  2pi Bound : Subsystem
  Demux : Demux  Outputs=3
  Mux : Mux  Inputs=3
  pi Bound : Subsystem
  pi/2 Bound : Subsystem
  Euler_bound : Outport
  wires:
  2pi Bound/1(Out) -> Mux/3
  Demux/3 -> 2pi Bound/1(In)
  Demux/2 -> pi Bound/1(In)
  Demux/1 -> pi/2 Bound/1(In)
  Euler_nobound/1 -> Demux/1
  Mux/1 -> Euler_bound/1
  pi/2 Bound/1(Out) -> Mux/1
  pi Bound/1(Out) -> Mux/2

== system SimCoreLib/Eom_Copy/Euler and DCM ==
  "p q r " : Inport
  DCM_321 : OpenFlightUtilLib/Transformations/DCM_321
  Demux3 : Demux  Outputs=3
  Euler Angle Bounds : Subsystem
  phi theta psi : Integrator  InitialCondition=Sim.Trim.Init.sInit_BL_rad  ContinuousStateAttributes='sState_BL_rad'
  phidot thetadot psidot : Subsystem
  Euler : Outport
  DCM : Outport  Port=2
  wires:
  Euler Angle Bounds/1(Euler_bound) -> Euler/1
  phi theta psi/1 -> phidot thetadot psidot/1(phi theta psi), Demux3/1, Euler Angle Bounds/1(Euler_nobound)
  phidot thetadot psidot/1(phidt thetadt psidt) -> phi theta psi/1
  "p q r "/1 -> phidot thetadot psidot/2(p q r)
  DCM_321/1 -> DCM/1
  Demux3/3 -> DCM_321/3
  Demux3/2 -> DCM_321/2
  Demux3/1 -> DCM_321/1

== system SimCoreLib/Eom_Copy/TransVelIntegration ==
  v_BE_L : Inport
  rInit_BE_D : Inport  Port=2
  Integrator : Integrator  ContinuousStateAttributes='rState_BE_L_m'
      settings: AttributesFormatString=State: %<ContinuousStateAttributes>
  Position2Geod : SimCoreLib/Position2Geod
  Sum2 : Sum  Inputs=|++
  r_BE_D : Outport
  r_BE_L : Outport  Port=2
  wires:
  rInit_BE_D/1 -> Sum2/2
  Sum2/1 -> r_BE_D/1  "r_BE_D_ddm"
  Integrator/1 -> Position2Geod/1, r_BE_L/1  "r_BE_L_m"
  Position2Geod/1 -> Sum2/1
  v_BE_L/1 -> Integrator/1

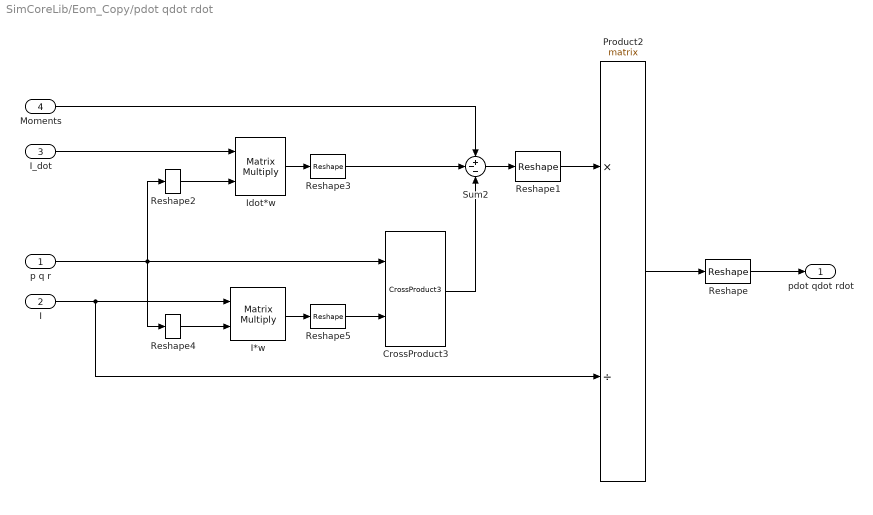
== system SimCoreLib/Eom_Copy/pdot qdot rdot ==
  p q r : Inport
  I : Inport  Port=2
  I_dot : Inport  Port=3
  Moments : Inport  Port=4
  CrossProduct3 : OpenFlightUtilLib/Math/CrossProduct3
  I*w : Product  Multiplication=Matrix(*)  SaturateOnIntegerOverflow=on  InputSameDT=on  OutDataTypeStr=Inherit: Same as first input
  Idot*w : Product  Multiplication=Matrix(*)  SaturateOnIntegerOverflow=on  InputSameDT=on  OutDataTypeStr=Inherit: Same as first input
  Product2 : Product  Inputs=*/  Multiplication=Matrix(*)  SaturateOnIntegerOverflow=on  OutDataTypeStr=Inherit: Same as first input
  Reshape : Reshape
  Reshape1 : Reshape  OutputDimensionality=Row vector (2-D)
  Reshape2 : Reshape  OutputDimensionality=Column vector (2-D)
  Reshape3 : Reshape
  Reshape4 : Reshape  OutputDimensionality=Column vector (2-D)
  Reshape5 : Reshape
  Sum2 : Sum  Inputs=+--  SaturateOnIntegerOverflow=on
  pdot qdot rdot : Outport
  wires:
  Reshape1/1 -> Product2/1
  Reshape5/1 -> CrossProduct3/2
  CrossProduct3/1 -> Sum2/3
  Reshape3/1 -> Sum2/2
  Moments/1 -> Sum2/1
  Sum2/1 -> Reshape1/1
  Product2/1 -> Reshape/1
  p q r/1 -> Reshape2/1, Reshape4/1, CrossProduct3/1
  Reshape/1 -> pdot qdot rdot/1
  Reshape2/1 -> Idot*w/2
  Idot*w/1 -> Reshape3/1
  I_dot/1 -> Idot*w/1
  Reshape4/1 -> I*w/2
  I/1 -> Product2/2, I*w/1
  I*w/1 -> Reshape5/1

== system SimCoreLib/Eom_LocalLevel/AngAccelIntegration ==
  note: w_BL_B = w_BI_B - w_EI_B - w_LE_B
      | w_EI_* = [0; 0; 0]; % Non-rotating Earth
      | w_LE_* = [0; 0; 0]; % Flat Earth
  note: wDot_BL_B = wDot_BI_B - wDot_EI_B - wDot_LE_B
      | wDot_EI_* = [0; 0; 0]; % By Definition
      | wDot_LE_* = [0; 0; 0]; % Flat Earth
  wDot_BI_B : Inport
  wGust_BI_B : Inport  Port=2
  Constant4 : Constant  Value=Sim.Trim.Init.wState_BI_B_rps
      settings: AttributesFormatString=%<Value>
  Gain : Gain
  Gain1 : Gain
  Integrator : Integrator  InitialConditionSource=external  ContinuousStateAttributes='wState_BI_B_rps'
      settings: AttributesFormatString=State: %<ContinuousStateAttributes>
  Sum2 : Sum  Inputs=|++  SaturateOnIntegerOverflow=on
  w_BL_B : Outport
  wDot_BL_B : Outport  Port=2
  w_BI_B : Outport  Port=3
  wires:
  Constant4/1 -> Integrator/2  "wInit_BI_B_rps"
  wGust_BI_B/1 -> Sum2/2
  Gain/1 -> wDot_BL_B/1  "wDot_BL_B_rps2"
  Gain1/1 -> w_BL_B/1  "w_BL_B_rps"
  wDot_BI_B/1 -> Gain/1, Integrator/1
  Integrator/1 -> Sum2/1  "w_BI_B_rps"
  Sum2/1 -> w_BI_B/1, Gain1/1  "w_BI_B_rps"

== system SimCoreLib/Eom_LocalLevel/AngVelIntegration_Quat ==
  w_BL_B : Inport
  Constant4 : Constant  Value=Sim.Trim.Init.quatState
      settings: AttributesFormatString=%<Value>
  NormL2 : OpenFlightUtilLib/Math/NormL2
  Product2 : Product  Inputs=*/  RndMeth=Zero
  Quat2DCM321 : OpenFlightUtilLib/Transformations/Quat2DCM
  Quat2Euler : OpenFlightUtilLib/Transformations/Quat2Euler
  QuatDeriv : OpenFlightUtilLib/Transformations/QuatDeriv
  QuatInt : OpenFlightUtilLib/Transformations/QuatInt
  T_L2B : Outport
  s_BL : Outport  Port=2
  wires:
  Quat2Euler/1 -> s_BL/1  "s_BL_rad"
  Quat2DCM321/1 -> T_L2B/1  "T_L2B"
  NormL2/1 -> Product2/2
  QuatDeriv/1 -> QuatInt/1  "quatDot_BL_nd"
  QuatInt/1 -> Product2/1, NormL2/1
  Product2/1 -> Quat2Euler/1, Quat2DCM321/1, QuatDeriv/1  "quat_BL_nd"
  Constant4/1 -> QuatInt/2  "quatInit_BL_nd"
  w_BL_B/1 -> QuatDeriv/2

== system SimCoreLib/Eom_LocalLevel/Force2Accel ==
  w_BI_B : Inport
  fExt : Inport  Port=2
  m : Inport  Port=3
  mDot : Inport  Port=4
  aGrav_BI_B : Inport  Port=5
  v_BI_B : Inport  Port=6
  Product : Product
  Sum2 : Sum  Inputs=|++  SaturateOnIntegerOverflow=on
  TransMomentumInv : OpenFlightUtilLib/Kinematics and Dynamics/TransMomentumInv
  m1 : InportShadow  Port=3
  a_BI_B : Outport
  wires:
  Sum2/1 -> TransMomentumInv/3  "aTot_BI_B_mps2"
  Product/1 -> Sum2/2
  m1/1 -> Product/1
  fExt/1 -> Sum2/1
  v_BI_B/1 -> TransMomentumInv/1
  w_BI_B/1 -> TransMomentumInv/5
  mDot/1 -> TransMomentumInv/4
  m/1 -> TransMomentumInv/2
  aGrav_BI_B/1 -> Product/2
  TransMomentumInv/1 -> a_BI_B/1  "a_BI_B_mps2"

== system SimCoreLib/Eom_LocalLevel/TransAccelIntegration ==
  a_BI_B : Inport
  T_B2I : Inport  Port=2
  vGust_BI_B : Inport  Port=3
  Constant4 : Constant  Value=Sim.Trim.Init.vState_BI_B_mps
      settings: AttributesFormatString=%<Value>
  Integrator : Integrator  InitialConditionSource=external  ContinuousStateAttributes='vState_BI_B_mps'
      settings: AttributesFormatString=State: %<ContinuousStateAttributes>
  Product1 : Product  Inputs=**  Multiplication=Matrix(*)  RndMeth=Zero
  Sum2 : Sum  Inputs=|++  SaturateOnIntegerOverflow=on
  v_BI_I : Outport
  v_BI_B : Outport  Port=2
  wires:
  Integrator/1 -> Sum2/1
  vGust_BI_B/1 -> Sum2/2
  Sum2/1 -> Product1/2, v_BI_B/1  "v_BI_B_mps"
  a_BI_B/1 -> Integrator/1
  T_B2I/1 -> Product1/1
  Product1/1 -> v_BI_I/1  "v_BI_I_mps"
  Constant4/1 -> Integrator/2  "vInit_BI_B_mps"

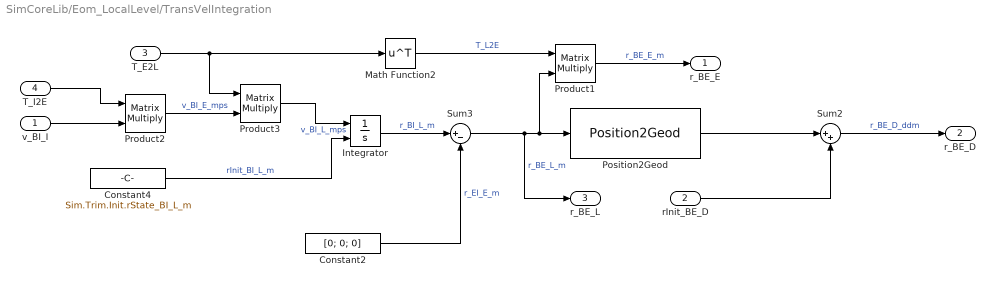
== system SimCoreLib/Eom_LocalLevel/TransVelIntegration ==
  v_BI_I : Inport
  rInit_BE_D : Inport  Port=2
  T_E2L : Inport  Port=3
  T_I2E : Inport  Port=4
  Constant2 : Constant  Value=[0; 0; 0]
      settings: AttributesFormatString=%<Value>
  Constant4 : Constant  Value=Sim.Trim.Init.rState_BI_L_m
      settings: AttributesFormatString=%<Value>
  Integrator : Integrator  InitialConditionSource=external  ContinuousStateAttributes='rState_BI_L_m'
      settings: AttributesFormatString=State: %<ContinuousStateAttributes>
  Math Function2 : Math  Operator=transpose  SaturateOnIntegerOverflow=on
  Position2Geod : SimCoreLib/Position2Geod
  Product1 : Product  Inputs=**  Multiplication=Matrix(*)  RndMeth=Zero
  Product2 : Product  Inputs=**  Multiplication=Matrix(*)  RndMeth=Zero
  Product3 : Product  Inputs=**  Multiplication=Matrix(*)  RndMeth=Zero
  Sum2 : Sum  Inputs=|++
  Sum3 : Sum  Inputs=|+-
  r_BE_E : Outport
  r_BE_D : Outport  Port=2
  r_BE_L : Outport  Port=3
  wires:
  Product1/1 -> r_BE_E/1  "r_BE_E_m"
  Math Function2/1 -> Product1/1  "T_L2E"
  Product3/1 -> Integrator/1  "v_BI_L_mps"
  Product2/1 -> Product3/2  "v_BI_E_mps"
  T_I2E/1 -> Product2/1
  Constant4/1 -> Integrator/2  "rInit_BI_L_m"
  Constant2/1 -> Sum3/2  "r_EI_E_m"
  Sum3/1 -> Position2Geod/1, Product1/2, r_BE_L/1  "r_BE_L_m"
  rInit_BE_D/1 -> Sum2/2
  Sum2/1 -> r_BE_D/1  "r_BE_D_ddm"
  T_E2L/1 -> Product3/1, Math Function2/1
  Position2Geod/1 -> Sum2/1
  Integrator/1 -> Sum3/1  "r_BI_L_m"
  v_BI_I/1 -> Product2/2

== system SimCoreLib/FlowConditions/ApplyWind ==
  note: aWind_BA_B = a_BI_B - a_EI_B - T_L2B * a_AE_L;
      |
      | a_EI_B = [0; 0; 0];
      | a_AE_L = aWind = 0; % Steady Wind
  note: vWind_BA_B = v_BE_B - T_L2B * v_AE_L;
      |
      | v_AE_L = vWind;
  Eom : Inport
  Env : Inport  Port=2
  Bus Selector1 : BusSelector  OutputSignals=v_BE_B_mps,T_L2B
  Bus Selector2 : BusSelector  OutputSignals=a_BI_B_mps2
  Bus Selector4 : BusSelector  OutputSignals=BusAtmos.vWind_mps
  Gain : Gain
  Product1 : Product  Inputs=**  Multiplication=Matrix(*)  RndMeth=Zero
  Sum1 : Sum  Inputs=|+-  SaturateOnIntegerOverflow=on
  v_BA_B : Outport
  a_BA_B : Outport  Port=2
  wires:
  Gain/1 -> a_BA_B/1  "a_BA_B_mps2"
  Bus Selector2/1 -> Gain/1  "<a_BI_B_mps2>"
  Sum1/1 -> v_BA_B/1  "v_BA_B_mps"
  Product1/1 -> Sum1/2  "v_AI_B_mps"
  Bus Selector1/2 -> Product1/1  "<T_L2B>"
  Bus Selector4/1 -> Product1/2  "<vWind_mps>"
  Bus Selector1/1 -> Sum1/1  "<v_BE_B_mps>"
  Eom/1 -> Bus Selector1/1, Bus Selector2/1
  Env/1 -> Bus Selector4/1

== system SimCoreLib/NavEquations/GeoidModel_EGM96 ==
  r_BI_D : Inport
  Demux2 : Demux  Outputs=3
  Look-Up Table (2-D) : Lookup2D  RowIndex=Sim.Nav.lat_deg  ColumnIndex=Sim.Nav.lon_deg  Table=Sim.Nav.altErr_m'  SaturateOnIntegerOverflow=on  InputSameDT=on
  Sum : Sum  Inputs=3
  WGS-84 correction : Constant  Value=Sim.Nav.wgs84Corr
  Alt MSL : Outport
  wires:
  WGS-84 correction/1 -> Sum/3
  Look-Up Table (2-D)/1 -> Sum/1
  Sum/1 -> Alt MSL/1
  Demux2/3 -> Sum/2
  r_BI_D/1 -> Demux2/1
  Demux2/1 -> Look-Up Table (2-D)/1
  Demux2/2 -> Look-Up Table (2-D)/2

== system SimCoreLib/NavEquations/Terrain ==
  Alt : Inport
  Alt Grnd : Inport  Port=2
  Sum : Sum  Inputs=|+-  SaturateOnIntegerOverflow=on  InputSameDT=on  OutDataTypeStr=Inherit: Same as first input
  Alt AGL : Outport
  wires:
  Alt/1 -> Sum/1
  Sum/1 -> Alt AGL/1  "altAgl_m"
  Alt Grnd/1 -> Sum/2

== system SimCoreLib/NavEquations/VelocityComposition ==
  note: Velocity Composition - NED
  v_BE_L : Inport
  Demux : Demux  Outputs=3
  Gain : Gain  Gain=-1
  Mux : Mux  Inputs=2
  NormL2 : OpenFlightUtilLib/Math/NormL2
  Trigonometric Function : Trigonometry  Operator=atan2
  Trigonometric Function1 : Trigonometry  Operator=atan2
  vGrnd (m/s) : Outport
  Flight Path Angle (rad) : Outport  Port=2
  Course (rad) : Outport  Port=3
  wires:
  Trigonometric Function1/1 -> Course (rad)/1
  Trigonometric Function/1 -> Flight Path Angle (rad)/1
  Mux/1 -> NormL2/1
  NormL2/1 -> vGrnd (m/s)/1, Trigonometric Function/2
  Gain/1 -> Trigonometric Function/1
  Demux/3 -> Gain/1
  Demux/2 -> Mux/2, Trigonometric Function1/1
  Demux/1 -> Trigonometric Function1/2, Mux/1
  v_BE_L/1 -> Demux/1

== system SimCoreLib/Eom_AeroBlock/Euler Angle Bounds/2pi Bound ==
  In : Inport
  2pi : Constant  Value=2*pi
  Math Function2 : Math  Operator=mod  SaturateOnIntegerOverflow=on
  Out : Outport
  wires:
  In/1 -> Math Function2/1
  2pi/1 -> Math Function2/2
  Math Function2/1 -> Out/1

== system SimCoreLib/Eom_AeroBlock/Euler Angle Bounds/pi Bound ==
  In : Inport
  Math Function1 : Math  Operator=mod  SaturateOnIntegerOverflow=on
  Sum3 : Sum  Inputs=|+-  SaturateOnIntegerOverflow=on  InputSameDT=on  OutDataTypeStr=Inherit: Same as first input
  Sum4 : Sum  Inputs=|++  SaturateOnIntegerOverflow=on  InputSameDT=on  OutDataTypeStr=Inherit: Same as first input
  pi2 : Constant  Value=pi
  pi3 : Constant  Value=2*pi
  Out : Outport
  wires:
  Sum3/1 -> Out/1
  pi2/1 -> Sum3/2, Sum4/2
  Sum4/1 -> Math Function1/1
  In/1 -> Sum4/1
  pi3/1 -> Math Function1/2
  Math Function1/1 -> Sum3/1

== system SimCoreLib/Eom_AeroBlock/Euler Angle Bounds/pi//2 Bound ==
  In : Inport
  Math Function : Math  Operator=mod  SaturateOnIntegerOverflow=on
  Sum1 : Sum  Inputs=|+-  SaturateOnIntegerOverflow=on  InputSameDT=on  OutDataTypeStr=Inherit: Same as first input
  Sum2 : Sum  Inputs=|++  SaturateOnIntegerOverflow=on  InputSameDT=on  OutDataTypeStr=Inherit: Same as first input
  pi : Constant  Value=pi/2
  pi1 : Constant  Value=pi
  Out : Outport
  wires:
  Math Function/1 -> Sum1/1
  pi1/1 -> Math Function/2
  In/1 -> Sum2/1
  Sum2/1 -> Math Function/1
  pi/1 -> Sum2/2, Sum1/2
  Sum1/1 -> Out/1

== system SimCoreLib/Eom_Copy/Euler and DCM/Euler Angle Bounds ==
  Euler_nobound : Inport
  2pi Bound : Subsystem
  Demux : Demux  Outputs=3
  Mux : Mux  Inputs=3
  pi Bound : Subsystem
  pi/2 Bound : Subsystem
  Euler_bound : Outport
  wires:
  pi Bound/1(Out) -> Mux/2
  pi/2 Bound/1(Out) -> Mux/1
  Mux/1 -> Euler_bound/1
  Euler_nobound/1 -> Demux/1
  Demux/1 -> pi/2 Bound/1(In)
  Demux/2 -> pi Bound/1(In)
  Demux/3 -> 2pi Bound/1(In)
  2pi Bound/1(Out) -> Mux/3

== system SimCoreLib/Eom_Copy/Euler and DCM/phidot thetadot psidot ==
  phi theta psi : Inport
  p q r : Inport  Port=2
  Mux1 : Mux  Inputs=[3 3]
  Mux4 : Mux  Inputs=3
  phi dot : Fcn  Expr=u(1)+(u(2)*sin(u(4))+u(3)*cos(u(4)))*tan(u(5))
  psi dot : Fcn  Expr=(u(2)*sin(u(4))+u(3)*cos(u(4)))/cos(u(5))
  theta dot : Fcn  Expr=u(2)*cos(u(4))-u(3)*sin(u(4))
  phidt thetadt psidt : Outport  InitialOutput=0
  wires:
  phi theta psi/1 -> Mux1/2
  Mux4/1 -> phidt thetadt psidt/1
  Mux1/1 -> psi dot/1, theta dot/1, phi dot/1
  phi dot/1 -> Mux4/1
  theta dot/1 -> Mux4/2
  psi dot/1 -> Mux4/3
  p q r/1 -> Mux1/1

== system SimCoreLib/Eom_Copy/Euler and DCM/Euler Angle Bounds/2pi Bound ==
  In : Inport
  2pi : Constant  Value=2*pi
  Math Function2 : Math  Operator=mod  SaturateOnIntegerOverflow=on
  Out : Outport
  wires:
  Math Function2/1 -> Out/1
  2pi/1 -> Math Function2/2
  In/1 -> Math Function2/1

== system SimCoreLib/Eom_Copy/Euler and DCM/Euler Angle Bounds/pi Bound ==
  In : Inport
  Math Function1 : Math  Operator=mod  SaturateOnIntegerOverflow=on
  Sum3 : Sum  Inputs=|+-  SaturateOnIntegerOverflow=on  InputSameDT=on  OutDataTypeStr=Inherit: Same as first input
  Sum4 : Sum  Inputs=|++  SaturateOnIntegerOverflow=on  InputSameDT=on  OutDataTypeStr=Inherit: Same as first input
  pi2 : Constant  Value=pi
  pi3 : Constant  Value=2*pi
  Out : Outport
  wires:
  Math Function1/1 -> Sum3/1
  pi3/1 -> Math Function1/2
  In/1 -> Sum4/1
  Sum4/1 -> Math Function1/1
  pi2/1 -> Sum4/2, Sum3/2
  Sum3/1 -> Out/1

== system SimCoreLib/Eom_Copy/Euler and DCM/Euler Angle Bounds/pi//2 Bound ==
  In : Inport
  Math Function : Math  Operator=mod  SaturateOnIntegerOverflow=on
  Sum1 : Sum  Inputs=|+-  SaturateOnIntegerOverflow=on  InputSameDT=on  OutDataTypeStr=Inherit: Same as first input
  Sum2 : Sum  Inputs=|++  SaturateOnIntegerOverflow=on  InputSameDT=on  OutDataTypeStr=Inherit: Same as first input
  pi : Constant  Value=pi/2
  pi1 : Constant  Value=pi
  Out : Outport
  wires:
  Sum1/1 -> Out/1
  pi/1 -> Sum1/2, Sum2/2
  Sum2/1 -> Math Function/1
  In/1 -> Sum2/1
  pi1/1 -> Math Function/2
  Math Function/1 -> Sum1/1
